simulink model "sim_0_1"  (R2021a)
settings: Solver=VariableStepAuto  StartTime=0.0  StopTime=2400  RelTol=1e-3
values from neighbouring files (symbols this model uses):
  A = 0.42    [variables.m]
  cd = 0.089    [variables.m]
  g = 9.81    [variables.m]
  m = 72    [variables.m]
  mi = 0.00082    [variables.m]
  R = 0.22    [variables.m]
  rho = 1.2    [variables.m]
libraries: pid_lib x1
settings Model: Creator=Adrian  LastModifiedBy=Adrian
settings SolverCC: ZeroCrossAlgorithm=Adaptive
settings DebuggingCC: IgnoredZcDiagnostic=none

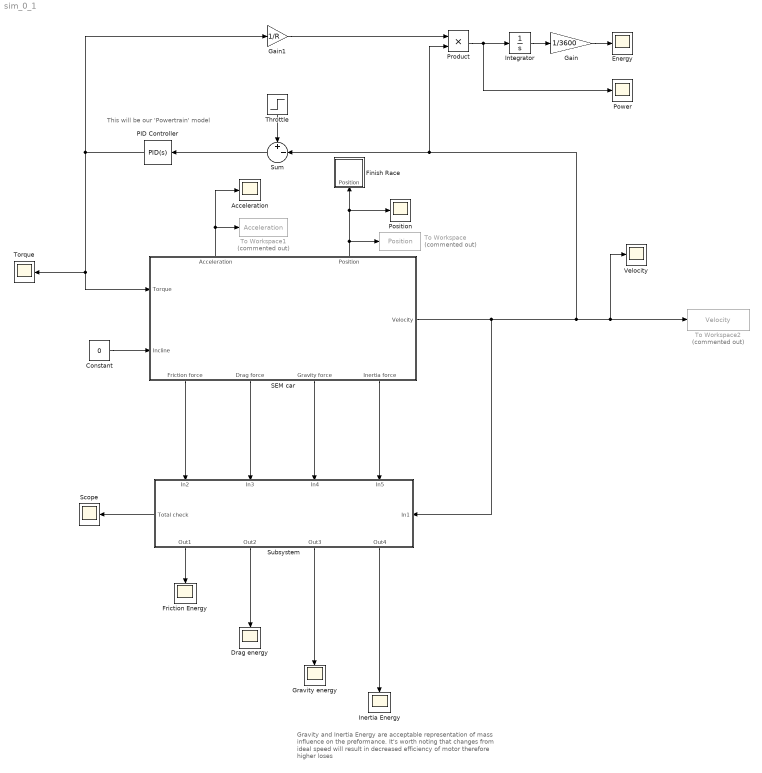
== system sim_0_1 ==
  note: Gravity and Inertia Energy are acceptable representation of mass influence on the preformance. It's worth noting that changes from ideal speed will result in decreased efficiency of motor therefore higher loses
  note: This will be our 'Powertrain' model
  Acceleration : Scope
  Constant : Constant  Value=0
  Drag energy : Scope
  Energy : Scope
  Finish Race : Subsystem  TreatAsAtomicUnit=on
  Friction Energy : Scope
  Gain : Gain  Gain=1/3600
  Gain1 : Gain  Gain=1/R
  Gravity energy : Scope
  Inertia Energy : Scope
  Integrator : Integrator
  PID Controller : pid_lib/PID Controller  Controller=PID  Form=Parallel  TimeDomain=Continuous-time  UseExternalTs=off  SampleTime=-1  IntegratorMethod=Forward Euler  FilterMethod=Forward Euler  ControllerParametersSource=internal  P=10  I=1  D=0  UseFilter=on  N=100  TunerSelectOption=Transfer Function Based (PID Tuner App)  InitialConditionSource=internal  InitialConditionForIntegrator=0  InitialConditionForFilter=0  DifferentiatorICPrevScaledInput=0  ExternalReset=none  TrackingMode=off  Kt=1  LimitOutput=off  SatLimitsSource=internal  UpperSaturationLimit=inf  LowerSaturationLimit=-inf  LinearizeAsGain=on  AntiWindupMode=none  Kb=1  POutMin=[]  POutMax=[]  IOutMin=[]  IOutMax=[]  DOutMin=[]  DOutMax=[]  NOutMin=[]  NOutMax=[]  SumOutMin=[]  SumOutMax=[]  SaturationOutMin=[]  SaturationOutMax=[]  PParamMin=[]  PParamMax=[]  IParamMin=[]  IParamMax=[]  DParamMin=[]  DParamMax=[]  NParamMin=[]  NParamMax=[]  KbParamMin=[]  KbParamMax=[]  KtParamMin=[]  KtParamMax=[]  KbOutMin=[]  KbOutMax=[]  KtOutMin=[]  KtOutMax=[]  IntegratorOutMin=[]  IntegratorOutMax=[]  FilterOutMin=[]  FilterOutMax=[]  SumI1OutMin=[]  SumI1OutMax=[]  SumI2OutMin=[]  SumI2OutMax=[]  SumI3OutMin=[]  SumI3OutMax=[]  SumI4OutMin=[]  SumI4OutMax=[]  SumDOutMin=[]  SumDOutMax=[]  DifferentiatorOutMin=[]  DifferentiatorOutMax=[]  FilterDiffOutCoefMin=[]  FilterDiffOutCoefMax=[]  ReciprocalOutMin=[]  ReciprocalOutMax=[]  SumDenOutMin=[]  SumDenOutMax=[]  SumNumOutMin=[]  SumNumOutMax=[]  DivideOutMin=[]  DivideOutMax=[]  UdiffTsProdOutMin=[]  UdiffTsProdOutMax=[]  NTsProdOutMin=[]  NTsProdOutMax=[]  UintegralTsProdOutMin=[]  UintegralTsProdOutMax=[]  UngainTsProdOutMin=[]  UngainTsProdOutMax=[]  IntegratorContinuousStateAttributes=''  IntegratorStateMustResolveToSignalObject=off  IntegratorRTWStateStorageClass=Auto  FilterContinuousStateAttributes=''  FilterStateMustResolveToSignalObject=off  FilterRTWStateStorageClass=Auto  ParallelPVariant=InternalParameters  IdealPVariant=Disabled  IVariant=InternalParameters  DVariant=InternalParameters  IntegratorVariant=Continuous  SatVariant=Disabled  AWVariant=Passthrough  PCopyVariant=Disabled  TRVariant=Disabled  FdbkBlocksVariant=Forward  IdealPFdbkVariant=Disabled  SatFdbkVariant=Disabled  DerivativeFilterVariant=ContFilter  NVariant=InternalParameters  NCopyVariant=Disabled  FilterICVariant=InternalICsFilter  IntegratorICVariant=InternalICs  ExternalResetVariant=Disabled  TRSumVariant=Passthrough  SumFdbkVariant=Disabled  SumVariant=Sum_PID  TsampFilterVariant=InternalTs  TsampNgainVariant=Passthrough  TsampIntegralVariant=Passthrough  ExternalSaturationOutDataTypeStr=Inherit: Same as second input
  Position : Scope
  Power : Scope
  Product : Product
  SEM car : Subsystem  TreatAsAtomicUnit=on
      settings: PortSchema="{\"entries\":[{\"content\":{\"sides\":[{\"content\":{\"connectorIds\":[\"In1\",\"In2\"]},\"type\":\"ConnectorPlacement.EquallySpacedRectSide\",\"uuid\":\"bc620abd-fd57-48f2-82c3-bc7c483b7b10\"},{\"content\":{\"connectorIds\":[\"Out1\"],\"side\":\"RIGHT\"},\"type\":\"ConnectorPlacement.EquallySpacedRectSide\",\"uuid\":\"18c7d919-a1df-4db2-a9bd-e56b0ea97514\"},{\"content\":{\"connectorIds\":[\"Out6\",\"Out7\"],\"side\":\"TOP\"},\"type\":\"ConnectorPlacement.EquallySpacedRectSide\",\"uuid\":\"00c1de2a-9064-45f1-8c7e-a72f8fca2129\"},{\"content\":{\"connectorIds\":[\"Out2\",\"Out3\",\"Out4\",\"Out5\"],\"side\":\"BOTTOM\"},\"type\":\"ConnectorPlacement.EquallySpacedRectSide\",\"uuid\":\"2c33daf5-7d38-4da5-8c34-0771ee13823f\"}]},\"type\":\"ConnectorPlacement.EquallySpacedConnector\",\"uuid\":\"9d8968ee-05d4-45d8-b464-688a26334e7a\"}],\"packageUris\":[\"http://schema.mathworks.com/mf0/Connector/R2020b\"],\"version\":\"1.0\"}"
  Scope : Scope
  Subsystem : Subsystem  TreatAsAtomicUnit=on
      settings: PortSchema="{\"entries\":[{\"content\":{\"sides\":[{\"content\":{\"connectorIds\":[\"In1\",\"In2\",\"In3\",\"In4\"]},\"type\":\"ConnectorPlacement.EquallySpacedRectSide\",\"uuid\":\"707fe713-01c2-4f56-9996-a906e0ef7602\"},{\"content\":{\"connectorIds\":[\"Out1\",\"Out2\",\"Out3\",\"Out4\"],\"side\":\"RIGHT\"},\"type\":\"ConnectorPlacement.EquallySpacedRectSide\",\"uuid\":\"a5a148d0-405d-40b9-9591-91290da25fd1\"},{\"content\":{\"connectorIds\":[\"Out5\"],\"side\":\"TOP\"},\"type\":\"ConnectorPlacement.EquallySpacedRectSide\",\"uuid\":\"8ebbdc3d-e27e-4ba5-b3ef-6603eee8791e\"},{\"content\":{\"connectorIds\":[\"In5\"],\"side\":\"BOTTOM\"},\"type\":\"ConnectorPlacement.EquallySpacedRectSide\",\"uuid\":\"bdc1ab5f-dab5-47d9-8df6-fb78c300adcf\"}]},\"type\":\"ConnectorPlacement.EquallySpacedConnector\",\"uuid\":\"3b9dfe39-2ecd-43ec-8eaa-138eb7b126d9\"}],\"packageUris\":[\"http://schema.mathworks.com/mf0/Connector/R2020b\"],\"version\":\"1.0\"}"
  Sum : Sum  Inputs=+-|
  Throttle : Step  After=7  SampleTime=0
  To Workspace : ToWorkspace  Commented=on  VariableName=Position  SaveFormat=Timeseries  SampleTime=-1
      settings: MaxDataPoints=1
  To Workspace1 : ToWorkspace  Commented=on  VariableName=Acceleration  SaveFormat=Timeseries  SampleTime=10
  To Workspace2 : ToWorkspace  Commented=on  VariableName=Velocity  SaveFormat=Timeseries  SampleTime=10
  Torque : Scope
  Velocity : Scope
  wires:
  PID Controller/1 -> Gain1/1, SEM car/1(Torque), Torque/1
  Constant/1 -> SEM car/2(Incline)
  SEM car/1(Velocity) -> Subsystem/5(In1), Product/2, Sum/2, Velocity/1, To Workspace2/1
  Sum/1 -> PID Controller/1
  Throttle/1 -> Sum/1
  Product/1 -> Power/1, Integrator/1
  Integrator/1 -> Gain/1
  Gain/1 -> Energy/1
  SEM car/6(Acceleration) -> To Workspace1/1, Acceleration/1
  SEM car/7(Position) -> To Workspace/1, Position/1, Finish Race/1(Position)
  SEM car/2(Friction force) -> Subsystem/1(In2)
  SEM car/3(Drag force) -> Subsystem/2(In3)
  SEM car/4(Gravity force) -> Subsystem/3(In4)
  SEM car/5(Inertia force) -> Subsystem/4(In5)
  Subsystem/1(Out1) -> Friction Energy/1
  Subsystem/2(Out2) -> Drag energy/1
  Subsystem/3(Out3) -> Gravity energy/1
  Subsystem/4(Out4) -> Inertia Energy/1
  Subsystem/5(Total check) -> Scope/1
  Gain1/1 -> Product/1

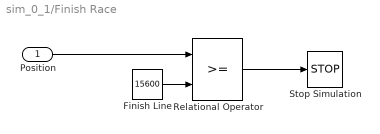
== system sim_0_1/Finish Race ==
  Position : Inport
  Finish Line : Constant  Value=15600
  Relational Operator : RelationalOperator  OutDataTypeStr=boolean  RndMeth=Simplest
  Stop Simulation : Stop
  wires:
  Finish Line/1 -> Relational Operator/2
  Relational Operator/1 -> Stop Simulation/1
  Position/1 -> Relational Operator/1

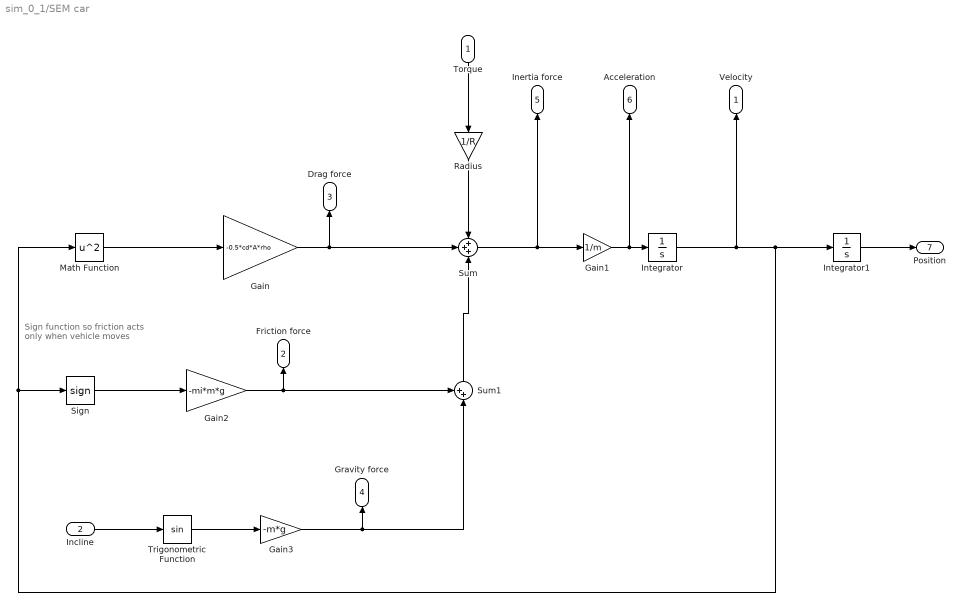
== system sim_0_1/SEM car ==
  note: Sign function so friction acts only when vehicle moves
  Torque : Inport
  Incline : Inport  Port=2
  Gain : Gain  Gain=-0.5*cd*A*rho
  Gain1 : Gain  Gain=1/m
  Gain2 : Gain  Gain=-mi*m*g
  Gain3 : Gain  Gain=-m*g
  Integrator : Integrator
  Integrator1 : Integrator
  Math Function : Math  Operator=square  SaturateOnIntegerOverflow=on
  Radius : Gain  Gain=1/R
  Sign : Signum
  Sum : Sum  Inputs=+++
  Sum1 : Sum  Inputs=++|
  Trigonometric Function : Trigonometry
  Velocity : Outport
  Friction force : Outport  Port=2
  Drag force : Outport  Port=3
  Gravity force : Outport  Port=4
  Inertia force : Outport  Port=5
  Acceleration : Outport  Port=6
  Position : Outport  Port=7
  wires:
  Sum/1 -> Gain1/1, Inertia force/1
  Math Function/1 -> Gain/1
  Integrator/1 -> Integrator1/1, Sign/1, Math Function/1, Velocity/1
  Torque/1 -> Radius/1
  Incline/1 -> Trigonometric Function/1
  Sum1/1 -> Sum/3
  Gain2/1 -> Friction force/1, Sum1/1
  Gain1/1 -> Acceleration/1, Integrator/1
  Integrator1/1 -> Position/1
  Gain3/1 -> Sum1/2, Gravity force/1
  Radius/1 -> Sum/1
  Gain/1 -> Sum/2, Drag force/1
  Trigonometric Function/1 -> Gain3/1
  Sign/1 -> Gain2/1

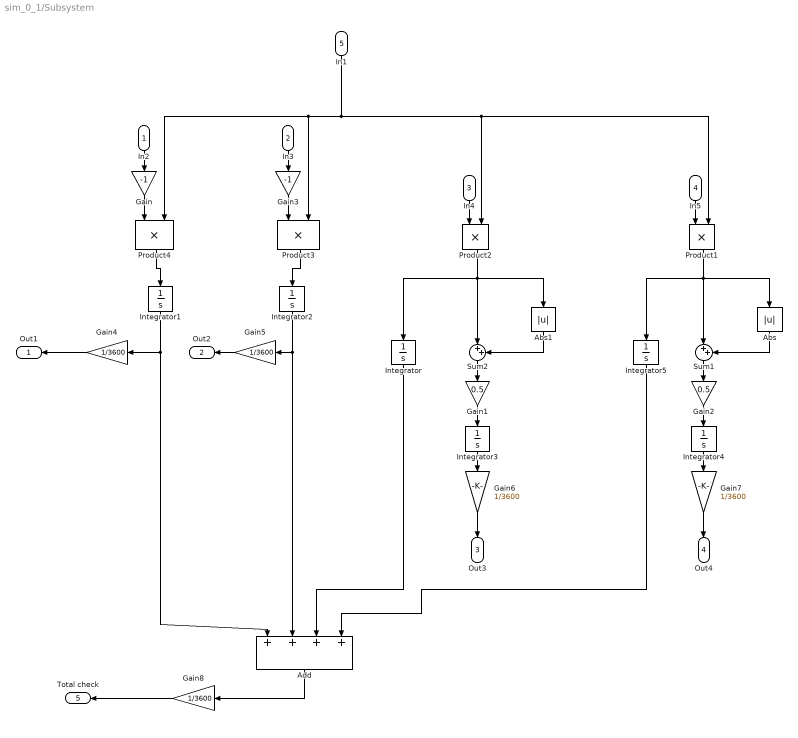
== system sim_0_1/Subsystem ==
  In2 : Inport
  In3 : Inport  Port=2
  In4 : Inport  Port=3
  In5 : Inport  Port=4
  In1 : Inport  Port=5
  Abs : Abs
  Abs1 : Abs
  Add : Sum  Inputs=++++
  Gain : Gain  Gain=-1
  Gain1 : Gain  Gain=0.5
  Gain2 : Gain  Gain=0.5
  Gain3 : Gain  Gain=-1
  Gain{4..8} (5 alike) : Gain  Gain=1/3600
  Integrator{,1..5} (6 alike) : Integrator
  Product{1..4} (4 alike) : Product
  Sum1 : Sum  Inputs=|++
  Sum2 : Sum  Inputs=|++
  Out1 : Outport
  Out2 : Outport  Port=2
  Out3 : Outport  Port=3
  Out4 : Outport  Port=4
  Total check : Outport  Port=5
  wires:
  Product4/1 -> Integrator1/1
  Gain1/1 -> Integrator3/1
  In1/1 -> Product4/2, Product3/2, Product1/2, Product2/2
  Product2/1 -> Integrator/1, Sum2/1, Abs1/1
  Abs1/1 -> Sum2/2
  Integrator1/1 -> Gain4/1, Add/1
  Sum1/1 -> Gain2/1
  Gain2/1 -> Integrator4/1
  Sum2/1 -> Gain1/1
  Product1/1 -> Integrator5/1, Sum1/1, Abs/1
  Product3/1 -> Integrator2/1
  In2/1 -> Gain/1
  Abs/1 -> Sum1/2
  In4/1 -> Product2/1
  In5/1 -> Product1/1
  Integrator2/1 -> Gain5/1, Add/2
  Integrator/1 -> Add/3
  Integrator5/1 -> Add/4
  Gain/1 -> Product4/1
  In3/1 -> Gain3/1
  Gain3/1 -> Product3/1
  Gain4/1 -> Out1/1
  Gain5/1 -> Out2/1
  Integrator3/1 -> Gain6/1
  Gain6/1 -> Out3/1
  Integrator4/1 -> Gain7/1
  Gain7/1 -> Out4/1
  Gain8/1 -> Total check/1
  Add/1 -> Gain8/1
